simulink model "matlab_fn_array_size"  (R2021a)
settings: Solver=VariableStepAuto  StartTime=0.0  StopTime=10.0  RelTol=1e-3
settings Model: Creator=Ms store  LastModifiedBy=Ms store

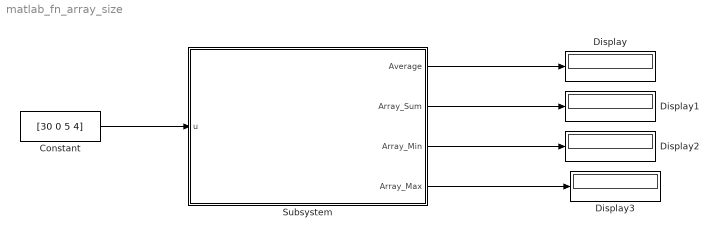
== system matlab_fn_array_size ==
  Constant : Constant  Value=[30 0 5 4]
  Display{,1..3} (4 alike) : Display
  Subsystem : Subsystem
  wires:
  Subsystem/1(Average) -> Display/1
  Subsystem/4(Array_Max) -> Display3/1
  Subsystem/3(Array_Min) -> Display2/1
  Subsystem/2(Array_Sum) -> Display1/1
  Constant/1 -> Subsystem/1(u)

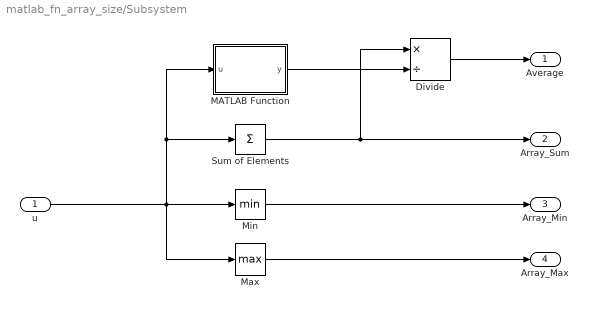
== system matlab_fn_array_size/Subsystem ==
  u : Inport
  Divide : Product  Inputs=*/
  MATLAB Function : MATLAB Function  TreatAsAtomicUnit=on
  Max : MinMax  Function=max
  Min : MinMax
  Sum of Elements : Sum  Inputs=+
  Average : Outport
  Array_Sum : Outport  Port=2
  Array_Min : Outport  Port=3
  Array_Max : Outport  Port=4
  wires:
  Sum of Elements/1 -> Divide/1, Array_Sum/1
  MATLAB Function/1(y) -> Divide/2
  Divide/1 -> Average/1
  Min/1 -> Array_Min/1
  Max/1 -> Array_Max/1
  u/1 -> MATLAB Function/1(u), Sum of Elements/1, Max/1, Min/1

== matlab function matlab_fn_array_size/Subsystem/MATLAB Function ==
  data: u input; y output
function y = Array_Size(u)

y = length(u);
